simulink model "controller"  (Simulink 8.3)
settings: Solver=FixedStepDiscrete  StartTime=0.0  StopTime=simulationTime  FixedStep=Ts  RelTol=1e-3
InitFcn:
  | initBalancingController_with_opt_of_tau;
values from neighbouring files (symbols this model uses):
  noOscillationTime = 0    [initBalancingController_with_opt_of_tau.m]    (also in initBalancingOptTau.m)
  number_of_feet_on_ground = 2    [initBalancingController_with_opt_of_tau.m]    (also in initBalancingOptTau.m)
  Ts = 0.01    [initBalancingController_with_opt_of_tau.m]    (also in initBalancingOptTau.m)
undefined symbols (not defined in the file or in its folder): amplitudesOscillationsOnOneFoot, dampings, directionOfOscillation, DiscIntNeverNeededParam, frequenciesOscillationsOnOneFoot, gainMomentum, gainsDCOM, gainsICOM, gainsPCOM, impedances, impedencesSat, increasingRatesImp, integralGains, qTildeMax, referenceParams, ROBOT_DOF, ROBOT_DOF_FOR_SIMULINK, satIntegral
undefined symbols (not defined in the file): localName, robotName
libraries: WBCLibrary x38
settings Model: Creator=daniele  LastModifiedBy=daniele
settings DataIOCC: SignalLoggingSaveFormat=Dataset
settings OptimizationCC: ExpressionDepthLimit=2147483647
settings DebuggingCC: FcnCallInpInsideContextMsg=EnableAllAsWarning
settings SFSimCC: SimParseCustomCode=off

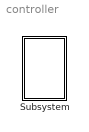
== system controller ==
  Subsystem : Subsystem  mask{robotName=robotName, Ts=Ts, localName=localName}
      mask prompts: robotName "robot name"; localName "module name"

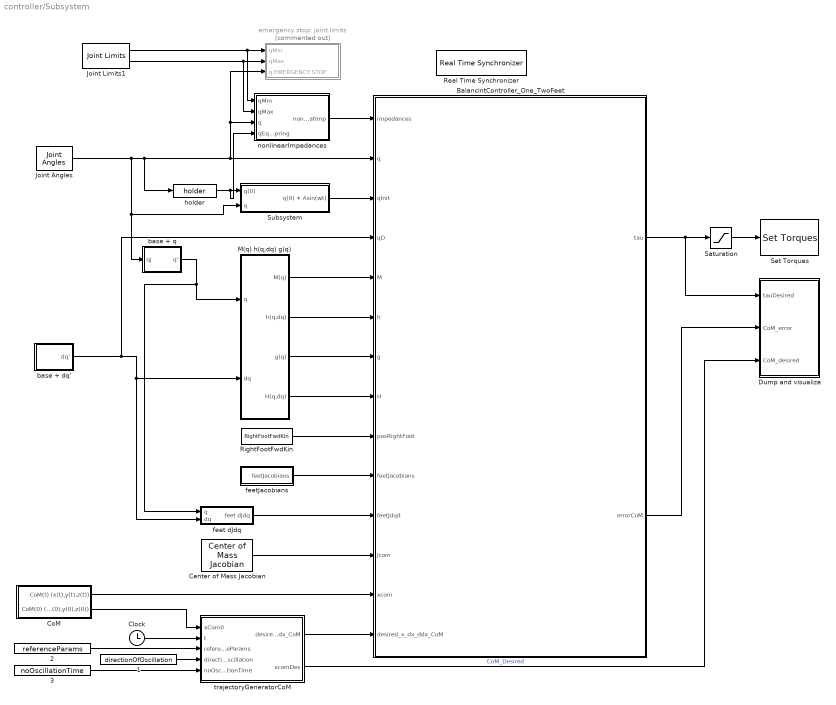
== system controller/Subsystem ==
  "    1" : Constant  Value=directionOfOscillation
  "    2" : Constant  Value=referenceParams
  "    3" : Constant  Value=noOscillationTime
  BalancintController_One_TwoFeet : Subsystem
  Center of Mass Jacobian : WBCLibrary/wholeBodyModel/Jacobians/Center of Mass Jacobian  robotName=robotName  localName=localName
  Clock : Clock
  "CoM " : Subsystem
  Dump and visualize : Subsystem
  Joint Angles : WBCLibrary/wholeBodyStates/Joint Angles  robotName=robotName  localName=localName
  Joint Limits1 : WBCLibrary/wholeBodyModel/Joint Limits  robotName=robotName  localName=localName
  M(q) h(q,dq) g(q) : Subsystem
  Real Time Synchronizer : WBCLibrary/Utilities/Real Time Synchronizer  Priority=-10  threadPeriod=Ts
  RightFootFwdKin : WBCLibrary/wholeBodyModel/Forward Kinematics/RightFootFwdKin  robotName=robotName  localName=localName
  Saturation : Saturate  UpperLimit=24  LowerLimit=-24
  Set Torques : WBCLibrary/wholeBodyActuators/Set Torques  val=6  robotName=robotName  localName=localName
  Subsystem : Subsystem
  base + dq' : Subsystem
  base + q : Subsystem
  emergency stop: joint limits : Subsystem  Commented=on
  feet dJdq : Subsystem
  feetJacobians : Subsystem
  "holder " : WBCLibrary/Utilities/holder 
  nonlinearImpedances : Subsystem
  trajectoryGeneratorCoM : MATLAB Function  TreatAsAtomicUnit=on
  wires:
  trajectoryGeneratorCoM/1(desired_x_dx_ddx_CoM) -> BalancintController_One_TwoFeet/14(desired_x_dx_ddx_CoM)
  "CoM "/2(CoM(0) (x(0),y(0),z(0))) -> trajectoryGeneratorCoM/1(xCom0)
  RightFootFwdKin/1 -> BalancintController_One_TwoFeet/9(posRightFoot)
  base + q/1(q') -> feet dJdq/1(q), M(q) h(q,dq) g(q)/1(q)
  M(q) h(q,dq) g(q)/3(g(q)) -> BalancintController_One_TwoFeet/7(g)
  M(q) h(q,dq) g(q)/4(H(q,dq)) -> BalancintController_One_TwoFeet/8(H)
  Center of Mass Jacobian/1 -> BalancintController_One_TwoFeet/12(Jcom)
  feetJacobians/1(feetJacobians) -> BalancintController_One_TwoFeet/10(feetJacobians)
  feet dJdq/1(feet dJdq) -> BalancintController_One_TwoFeet/11(feetJdqd)
  "holder "/1 -> nonlinearImpedances/4(qEquSpring), Subsystem/1(q(0))
  "CoM "/1(CoM(t) (x(t),y(t),z(t))) -> BalancintController_One_TwoFeet/13(xcom)
  base + dq'/1(dq') -> BalancintController_One_TwoFeet/4(qD), feet dJdq/2(dq), M(q) h(q,dq) g(q)/2(dq)
  M(q) h(q,dq) g(q)/1(M(q)) -> BalancintController_One_TwoFeet/5(M)
  M(q) h(q,dq) g(q)/2(h(q,dq)) -> BalancintController_One_TwoFeet/6(h)
  BalancintController_One_TwoFeet/1(tau) -> Saturation/1, Dump and visualize/1(tauDesired)
  "    2"/1 -> trajectoryGeneratorCoM/3(referenceParams)
  Clock/1 -> trajectoryGeneratorCoM/2(t)
  nonlinearImpedances/1(nonLinSatImp) -> BalancintController_One_TwoFeet/1(impedances)
  Joint Limits1/1 -> emergency stop: joint limits/1(qMin), nonlinearImpedances/1(qMin)
  Joint Limits1/2 -> emergency stop: joint limits/2(qMax), nonlinearImpedances/2(qMax)
  Joint Angles/1 -> Subsystem/2(q), base + q/1(qj), nonlinearImpedances/3(q), emergency stop: joint limits/3(q EMERGENCY STOP), BalancintController_One_TwoFeet/2(q), "holder "/1
  "    1"/1 -> trajectoryGeneratorCoM/4(directionOfOscillation)
  "    3"/1 -> trajectoryGeneratorCoM/5(noOscillationTime)
  Subsystem/1(q(0) + Asin(wt)) -> BalancintController_One_TwoFeet/3(qInit)
  BalancintController_One_TwoFeet/2(errorCoM) -> Dump and visualize/2(CoM_error)
  trajectoryGeneratorCoM/2(xcomDes) -> Dump and visualize/3(CoM_desired)  "CoM_Desired"
  Saturation/1 -> Set Torques/1

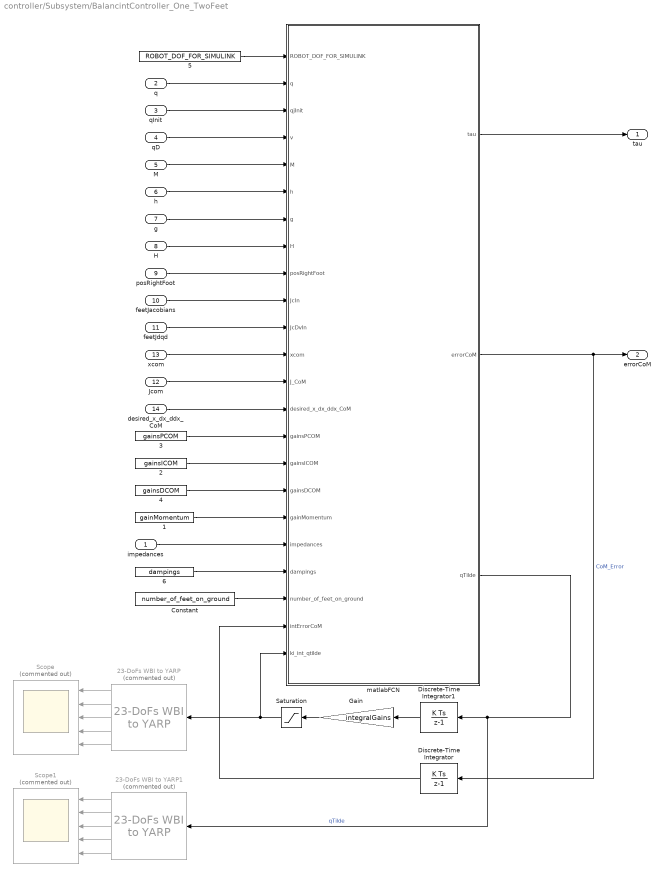
== system controller/Subsystem/BalancintController_One_TwoFeet ==
  impedances : Inport
  q : Inport  Port=2
  qInit : Inport  Port=3
  qD : Inport  Port=4
  M : Inport  Port=5
  h : Inport  Port=6
  g : Inport  Port=7
  H : Inport  Port=8
  posRightFoot : Inport  Port=9
  feetJacobians : Inport  Port=10
  feetJdqd : Inport  Port=11
  Jcom : Inport  Port=12
  xcom : Inport  Port=13
  desired_x_dx_ddx_CoM : Inport  Port=14
  "    1" : Constant  Value=gainMomentum
  "    2" : Constant  Value=gainsICOM
  "    3" : Constant  Value=gainsPCOM
  "    4" : Constant  Value=gainsDCOM
  "    5" : Constant  Value=ROBOT_DOF_FOR_SIMULINK
  "    6" : Constant  Value=dampings
  23-DoFs WBI to YARP : WBCLibrary/Utilities/23-DoFs WBI to YARP  Commented=on
  23-DoFs WBI to YARP1 : WBCLibrary/Utilities/23-DoFs WBI to YARP  Commented=on
  Constant : Constant  Value=number_of_feet_on_ground
  Discrete-Time Integrator : DiscreteIntegrator  InitialCondition=[0 0 0]  SampleTime=Ts  ICPrevOutput=DiscIntNeverNeededParam  ICPrevScaledInput=DiscIntNeverNeededParam
  Discrete-Time Integrator1 : DiscreteIntegrator  InitialCondition=zeros(ROBOT_DOF,1)  SampleTime=Ts  ICPrevOutput=DiscIntNeverNeededParam  ICPrevScaledInput=DiscIntNeverNeededParam
  Gain : Gain  Gain=integralGains
  Saturation : Saturate  UpperLimit=satIntegral  LowerLimit=-satIntegral
  Scope : Scope  Commented=on  NumInputPorts=5
      settings: ShowLegends=on  YMin=-5~-5~-5~-5~-5  YMax=5~5~5~5~5
  Scope1 : Scope  Commented=on  NumInputPorts=5
      settings: ShowLegends=on  YMin=-5~-5~-5~-5~-5  YMax=5~5~5~5~5  SaveName=ScopeData2
  matlabFCN : MATLAB Function  TreatAsAtomicUnit=on
  tau : Outport
  errorCoM : Outport  Port=2
  wires:
  q/1 -> matlabFCN/2(q)
  qInit/1 -> matlabFCN/3(qjInit)
  qD/1 -> matlabFCN/4(v)
  M/1 -> matlabFCN/5(M)
  h/1 -> matlabFCN/6(h)
  g/1 -> matlabFCN/7(g)
  H/1 -> matlabFCN/8(H)
  posRightFoot/1 -> matlabFCN/9(posRightFoot)
  feetJacobians/1 -> matlabFCN/10(JcIn)
  feetJdqd/1 -> matlabFCN/11(JcDvIn)
  xcom/1 -> matlabFCN/12(xcom)
  Jcom/1 -> matlabFCN/13(J_CoM)
  desired_x_dx_ddx_CoM/1 -> matlabFCN/14(desired_x_dx_ddx_CoM)
  impedances/1 -> matlabFCN/19(impedances)
  "    3"/1 -> matlabFCN/15(gainsPCOM)
  "    1"/1 -> matlabFCN/18(gainMomentum)
  "    2"/1 -> matlabFCN/16(gainsICOM)
  "    4"/1 -> matlabFCN/17(gainsDCOM)
  matlabFCN/1(tau) -> tau/1
  Constant/1 -> matlabFCN/21(number_of_feet_on_ground)
  "    5"/1 -> matlabFCN/1(ROBOT_DOF_FOR_SIMULINK)
  "    6"/1 -> matlabFCN/20(dampings)
  Discrete-Time Integrator/1 -> matlabFCN/22(intErrorCoM)
  matlabFCN/2(errorCoM) -> errorCoM/1, Discrete-Time Integrator/1  "CoM_Error"
  Discrete-Time Integrator1/1 -> Gain/1
  23-DoFs WBI to YARP/5 -> Scope/5
  23-DoFs WBI to YARP/1 -> Scope/1
  23-DoFs WBI to YARP/4 -> Scope/4
  23-DoFs WBI to YARP/2 -> Scope/2
  23-DoFs WBI to YARP/3 -> Scope/3
  matlabFCN/3(qTilde) -> 23-DoFs WBI to YARP1/1, Discrete-Time Integrator1/1  "qTilde"
  Gain/1 -> Saturation/1
  Saturation/1 -> 23-DoFs WBI to YARP/1, matlabFCN/23(ki_int_qtilde)
  23-DoFs WBI to YARP1/5 -> Scope1/5
  23-DoFs WBI to YARP1/1 -> Scope1/1
  23-DoFs WBI to YARP1/4 -> Scope1/4
  23-DoFs WBI to YARP1/2 -> Scope1/2
  23-DoFs WBI to YARP1/3 -> Scope1/3

== system controller/Subsystem/CoM  ==
  "COMFwdKin " : WBCLibrary/wholeBodyModel/Forward Kinematics/COMFwdKin   robotName=robotName  localName=localName
  "CoM6D ->  CoMXYZ" : Selector  InputPortWidth=7  Indices=[1 2 3]
  "holder " : WBCLibrary/Utilities/holder 
  CoM(t) (x(t),y(t),z(t)) : Outport
  CoM(0) (x(0),y(0),z(0)) : Outport  Port=2
  wires:
  "COMFwdKin "/1 -> "CoM6D ->  CoMXYZ"/1
  "CoM6D ->  CoMXYZ"/1 -> "holder "/1, CoM(t) (x(t),y(t),z(t))/1
  "holder "/1 -> CoM(0) (x(0),y(0),z(0))/1

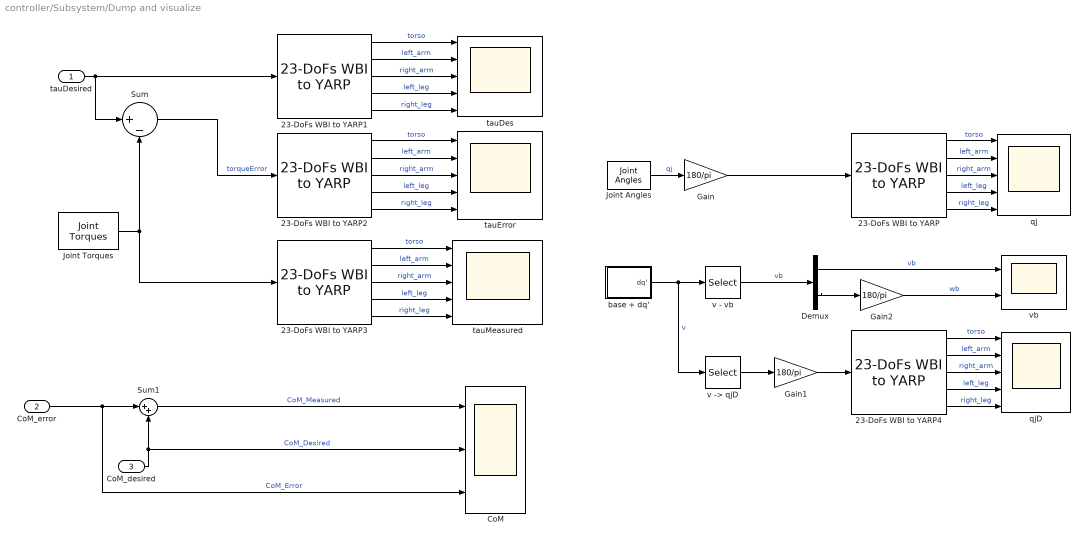
== system controller/Subsystem/Dump and visualize ==
  tauDesired : Inport
  CoM_error : Inport  Port=2
  CoM_desired : Inport  Port=3
  23-DoFs WBI to YARP{,1..4} (5 alike) : WBCLibrary/Utilities/23-DoFs WBI to YARP
  CoM : Scope  NumInputPorts=3
      settings: ShowLegends=on  TimeRange=400  YMin=-0.2~-0.2~-0.006  YMax=0.5~0.5~0.004  SaveName=CoM_data
  Demux : Demux  Outputs=2
  Gain : Gain  Gain=180/pi
  Gain1 : Gain  Gain=180/pi
  Gain2 : Gain  Gain=180/pi
  Joint Angles : WBCLibrary/wholeBodyStates/Joint Angles  robotName=robotName  localName=localName
  Joint Torques : WBCLibrary/wholeBodyStates/Joint Torques  robotName=robotName  localName=localName
  Sum : Sum  Inputs=|+-
  Sum1 : Sum  Inputs=|++
  base + dq' : Subsystem
  qj : Scope  NumInputPorts=5
      settings: ShowLegends=on  TimeRange=40  YMin=-10~-50~-50~-20~-40  YMax=10~100~100~40~40  SaveName=qj_and_v
  qjD : Scope  NumInputPorts=5
      settings: ShowLegends=on  TimeRange=40  YMin=-15~-10~-20~-20~-20  YMax=20~10~30~20~20  SaveName=qj_and_v1
  tauDes : Scope  NumInputPorts=5
      settings: ShowLegends=on  TimeRange=14  YMin=-20~-3~-3~-8~-10  YMax=10~3~3~4~10  SaveName=tauDes
  tauError : Scope  NumInputPorts=5
      settings: ShowLegends=on  TimeRange=90  YMin=-3~-6~-5~-4~-4  YMax=3~6~5~4~6  SaveName=tauError
  tauMeasured : Scope  NumInputPorts=5
      settings: ShowLegends=on  TimeRange=14  YMin=-15~-8~-5~-8~-10  YMax=10~4~5~6~10  SaveName=tauMeasured
  v - vb : Selector  InputPortWidth=ROBOT_DOF+6  Indices=[1:6]
  "v -> qjD" : Selector  InputPortWidth=ROBOT_DOF+6  Indices=[7:ROBOT_DOF+6]
  vb : Scope  NumInputPorts=2
      settings: ShowLegends=on  TimeRange=40  YMin=-0.08~-10  YMax=0.08~10  SaveName=qj_and_v2
  wires:
  CoM_error/1 -> CoM/3, Sum1/1  "CoM_Error"
  tauDesired/1 -> Sum/1, 23-DoFs WBI to YARP1/1
  Joint Torques/1 -> 23-DoFs WBI to YARP3/1, Sum/2
  CoM_desired/1 -> Sum1/2, CoM/2  "CoM_Desired"
  Sum1/1 -> CoM/1  "CoM_Measured"
  base + dq'/1(dq') -> "v -> qjD"/1, v - vb/1  "v"
  Joint Angles/1 -> Gain/1  "qj"
  Gain/1 -> 23-DoFs WBI to YARP/1
  23-DoFs WBI to YARP/5 -> qj/5  "right_leg"
  23-DoFs WBI to YARP/1 -> qj/1  "torso"
  23-DoFs WBI to YARP/2 -> qj/2  "left_arm"
  23-DoFs WBI to YARP/4 -> qj/4  "left_leg"
  23-DoFs WBI to YARP/3 -> qj/3  "right_arm"
  23-DoFs WBI to YARP1/5 -> tauDes/5  "right_leg"
  23-DoFs WBI to YARP1/1 -> tauDes/1  "torso"
  23-DoFs WBI to YARP1/2 -> tauDes/2  "left_arm"
  23-DoFs WBI to YARP1/4 -> tauDes/4  "left_leg"
  23-DoFs WBI to YARP1/3 -> tauDes/3  "right_arm"
  23-DoFs WBI to YARP2/5 -> tauError/5  "right_leg"
  23-DoFs WBI to YARP2/1 -> tauError/1  "torso"
  23-DoFs WBI to YARP2/2 -> tauError/2  "left_arm"
  23-DoFs WBI to YARP2/4 -> tauError/4  "left_leg"
  23-DoFs WBI to YARP2/3 -> tauError/3  "right_arm"
  Sum/1 -> 23-DoFs WBI to YARP2/1  "torqueError"
  23-DoFs WBI to YARP3/5 -> tauMeasured/5  "right_leg"
  23-DoFs WBI to YARP3/1 -> tauMeasured/1  "torso"
  23-DoFs WBI to YARP3/2 -> tauMeasured/2  "left_arm"
  23-DoFs WBI to YARP3/4 -> tauMeasured/4  "left_leg"
  23-DoFs WBI to YARP3/3 -> tauMeasured/3  "right_arm"
  23-DoFs WBI to YARP4/5 -> qjD/5  "right_leg"
  23-DoFs WBI to YARP4/1 -> qjD/1  "torso"
  23-DoFs WBI to YARP4/2 -> qjD/2  "left_arm"
  23-DoFs WBI to YARP4/4 -> qjD/4  "left_leg"
  23-DoFs WBI to YARP4/3 -> qjD/3  "right_arm"
  "v -> qjD"/1 -> Gain1/1
  v - vb/1 -> Demux/1  "vb"
  Demux/1 -> vb/1  "vb"
  Demux/2 -> Gain2/1
  Gain1/1 -> 23-DoFs WBI to YARP4/1
  Gain2/1 -> vb/2  "wb"

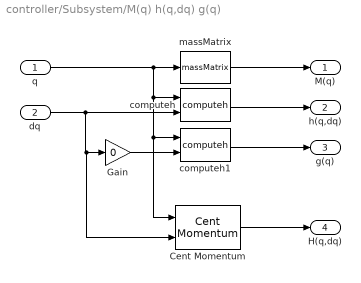
== system controller/Subsystem/M(q) h(q,dq) g(q) ==
  q : Inport
  dq : Inport  Port=2
  Cent Momentum : WBCLibrary/wholeBodyModel/Dynamics/Cent Momentum  robotName=robotName  localName=localName
  Gain : Gain  Gain=0
  computeh : WBCLibrary/wholeBodyModel/Dynamics/computeh  val=7  robotname=robotName  localname=localName
  computeh1 : WBCLibrary/wholeBodyModel/Dynamics/computeh  val=7  robotname=robotName  localname=localName
  massMatrix : WBCLibrary/wholeBodyModel/Dynamics/massMatrix  val=8  robotname=robotName  localname=localName
  M(q) : Outport
  h(q,dq) : Outport  Port=2
  g(q) : Outport  Port=3
  H(q,dq) : Outport  Port=4
  wires:
  Gain/1 -> computeh1/2
  computeh1/1 -> g(q)/1
  computeh/1 -> h(q,dq)/1
  massMatrix/1 -> M(q)/1
  q/1 -> Cent Momentum/1, computeh1/1, computeh/1, massMatrix/1
  dq/1 -> Cent Momentum/2, Gain/1, computeh/2
  Cent Momentum/1 -> H(q,dq)/1

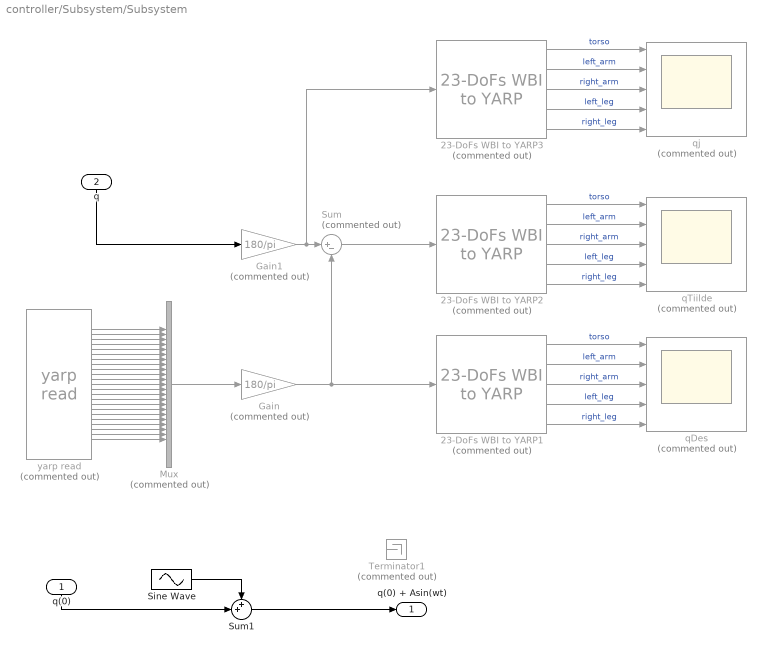
== system controller/Subsystem/Subsystem ==
  q(0) : Inport
  q : Inport  Port=2
  23-DoFs WBI to YARP1 : WBCLibrary/Utilities/23-DoFs WBI to YARP  Commented=on
  23-DoFs WBI to YARP2 : WBCLibrary/Utilities/23-DoFs WBI to YARP  Commented=on
  23-DoFs WBI to YARP3 : WBCLibrary/Utilities/23-DoFs WBI to YARP  Commented=on
  Gain : Gain  Commented=on  Gain=180/pi
  Gain1 : Gain  Commented=on  Gain=180/pi
  Mux : Mux  Commented=on  Inputs=23
  Sine Wave : Sin  Amplitude=amplitudesOscillationsOnOneFoot*pi/180  Frequency=frequenciesOscillationsOnOneFoot*2*pi  SampleTime=0
  Sum : Sum  Commented=on  Inputs=|+-
  Sum1 : Sum  Inputs=++|
  Terminator1 : Terminator  Commented=on
  qDes : Scope  Commented=on  NumInputPorts=5
      settings: ShowLegends=on  TimeRange=14  YMin=-20~-4~-4~-8~-10  YMax=10~4~4~4~10  SaveName=tauDes1
  qTiilde : Scope  Commented=on  NumInputPorts=5
      settings: ShowLegends=on  TimeRange=14  YMin=-20~-4~-4~-8~-10  YMax=10~4~4~4~10  SaveName=tauDes2
  qj : Scope  Commented=on  NumInputPorts=5
      settings: ShowLegends=on  TimeRange=14  YMin=-20~-4~-4~-8~-10  YMax=10~4~4~4~10  SaveName=tauDes3
  yarp read : WBCLibrary/Utilities/yarp read  Commented=on  from=['/trajGenY2/qdes:o']  to='...'  num=23  blocking=off  timestamp=off  autoconnect=on
  q(0) + Asin(wt) : Outport
  wires:
  q(0)/1 -> Sum1/2
  Sine Wave/1 -> Sum1/1
  Mux/1 -> Gain/1
  Gain/1 -> 23-DoFs WBI to YARP1/1, Sum/2
  q/1 -> Gain1/1
  Sum/1 -> 23-DoFs WBI to YARP2/1
  yarp read/18 -> Mux/18
  yarp read/16 -> Mux/16
  yarp read/21 -> Mux/21
  yarp read/23 -> Mux/23
  yarp read/22 -> Mux/22
  yarp read/17 -> Mux/17
  yarp read/19 -> Mux/19
  yarp read/20 -> Mux/20
  yarp read/4 -> Mux/4
  yarp read/5 -> Mux/5
  yarp read/6 -> Mux/6
  yarp read/7 -> Mux/7
  yarp read/8 -> Mux/8
  yarp read/9 -> Mux/9
  yarp read/10 -> Mux/10
  yarp read/11 -> Mux/11
  yarp read/12 -> Mux/12
  yarp read/13 -> Mux/13
  yarp read/14 -> Mux/14
  yarp read/3 -> Mux/3
  yarp read/1 -> Mux/1
  yarp read/2 -> Mux/2
  yarp read/15 -> Mux/15
  Gain1/1 -> 23-DoFs WBI to YARP3/1, Sum/1
  23-DoFs WBI to YARP1/5 -> qDes/5  "right_leg"
  23-DoFs WBI to YARP1/1 -> qDes/1  "torso"
  23-DoFs WBI to YARP1/2 -> qDes/2  "left_arm"
  23-DoFs WBI to YARP1/4 -> qDes/4  "left_leg"
  23-DoFs WBI to YARP1/3 -> qDes/3  "right_arm"
  23-DoFs WBI to YARP2/5 -> qTiilde/5  "right_leg"
  23-DoFs WBI to YARP2/1 -> qTiilde/1  "torso"
  23-DoFs WBI to YARP2/2 -> qTiilde/2  "left_arm"
  23-DoFs WBI to YARP2/4 -> qTiilde/4  "left_leg"
  23-DoFs WBI to YARP2/3 -> qTiilde/3  "right_arm"
  23-DoFs WBI to YARP3/5 -> qj/5  "right_leg"
  23-DoFs WBI to YARP3/1 -> qj/1  "torso"
  23-DoFs WBI to YARP3/2 -> qj/2  "left_arm"
  23-DoFs WBI to YARP3/4 -> qj/4  "left_leg"
  23-DoFs WBI to YARP3/3 -> qj/3  "right_arm"
  Sum1/1 -> q(0) + Asin(wt)/1

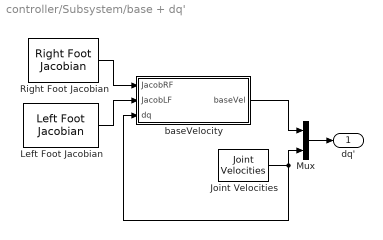
== system controller/Subsystem/base + dq' ==
  Joint Velocities : WBCLibrary/wholeBodyStates/Joint Velocities  robotName=robotName  localName=localName
  Left Foot Jacobian : WBCLibrary/wholeBodyModel/Jacobians/Left Foot Jacobian  robotName=robotName  localName=localName
  Mux : Mux  Inputs=2
  Right Foot Jacobian : WBCLibrary/wholeBodyModel/Jacobians/Right Foot Jacobian  robotName=robotName  localName=localName
  baseVelocity : Subsystem  AncestorBlock=WBCLibrary/Utilities/baseVelocity  mask(baseVelocity){}
      mask help: This block computes the velocity of the floating base of a bipedal robot
  dq' : Outport
  wires:
  Left Foot Jacobian/1 -> baseVelocity/2(JacobLF)
  Right Foot Jacobian/1 -> baseVelocity/1(JacobRF)
  baseVelocity/1(baseVel) -> Mux/1
  Joint Velocities/1 -> baseVelocity/3(dq), Mux/2
  Mux/1 -> dq'/1

== system controller/Subsystem/base + q ==
  qj : Inport
  Constant1 : Constant  Value=zeros(16,1)
  Mux : Mux  Inputs=2
  q' : Outport
  wires:
  Mux/1 -> q'/1
  qj/1 -> Mux/2
  Constant1/1 -> Mux/1

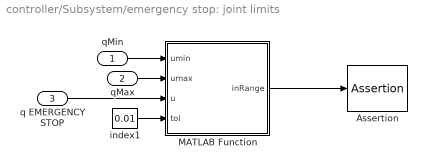
== system controller/Subsystem/emergency stop: joint limits ==
  qMin : Inport
  qMax : Inport  Port=2
  q EMERGENCY STOP : Inport  Port=3
  Assertion : Assertion
  MATLAB Function : MATLAB Function  TreatAsAtomicUnit=on
  index1 : Constant  Value=0.01  VectorParams1D=off
  wires:
  qMin/1 -> MATLAB Function/1(umin)
  qMax/1 -> MATLAB Function/2(umax)
  index1/1 -> MATLAB Function/4(tol)
  q EMERGENCY STOP/1 -> MATLAB Function/3(u)
  MATLAB Function/1(inRange) -> Assertion/1

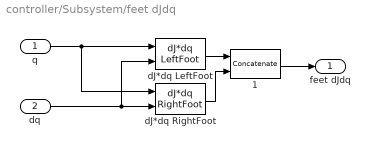
== system controller/Subsystem/feet dJdq ==
  q : Inport
  dq : Inport  Port=2
  " 1" : Concatenate  Mode=Multidimensional array
  dJ*dq LeftFoot : WBCLibrary/wholeBodyModel/Dynamics/dJ*dq LeftFoot  val=9  robotName=robotName  localName=localName
  dJ*dq RightFoot : WBCLibrary/wholeBodyModel/Dynamics/dJ*dq RightFoot  val=9  robotName=robotName  localName=localName
  feet dJdq : Outport
  wires:
  dJ*dq LeftFoot/1 -> " 1"/1
  dJ*dq RightFoot/1 -> " 1"/2
  " 1"/1 -> feet dJdq/1
  q/1 -> dJ*dq RightFoot/1, dJ*dq LeftFoot/1
  dq/1 -> dJ*dq LeftFoot/2, dJ*dq RightFoot/2

== system controller/Subsystem/feetJacobians ==
  " " : Concatenate  Mode=Multidimensional array
  Left Foot Jacobian : WBCLibrary/wholeBodyModel/Jacobians/Left Foot Jacobian  robotName=robotName  localName=localName
  Right Foot Jacobian : WBCLibrary/wholeBodyModel/Jacobians/Right Foot Jacobian  robotName=robotName  localName=localName
  feetJacobians : Outport
  wires:
  Left Foot Jacobian/1 -> " "/1
  Right Foot Jacobian/1 -> " "/2
  " "/1 -> feetJacobians/1

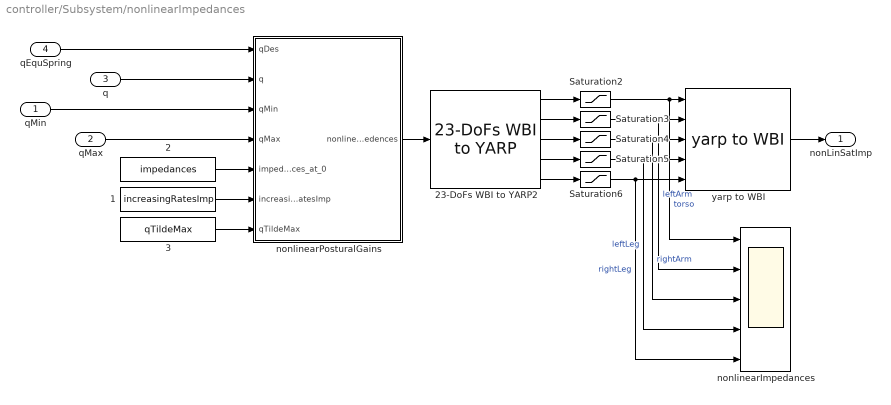
== system controller/Subsystem/nonlinearImpedances ==
  qMin : Inport
  qMax : Inport  Port=2
  q : Inport  Port=3
  qEquSpring : Inport  Port=4
  "    1" : Constant  Value=increasingRatesImp
  "    2" : Constant  Value=impedances
  "    3" : Constant  Value=qTildeMax
  23-DoFs WBI to YARP2 : WBCLibrary/Utilities/23-DoFs WBI to YARP
  Saturation2 : Saturate  UpperLimit=impedencesSat(1)  LowerLimit=0  SampleTime=Ts
  Saturation3 : Saturate  UpperLimit=impedencesSat(2)  LowerLimit=0  SampleTime=Ts
  Saturation4 : Saturate  UpperLimit=impedencesSat(2)  LowerLimit=0  SampleTime=Ts
  Saturation5 : Saturate  UpperLimit=impedencesSat(3)  LowerLimit=0  SampleTime=Ts
  Saturation6 : Saturate  UpperLimit=impedencesSat(3)  LowerLimit=0  SampleTime=Ts
  nonlinearImpedances : Scope  NumInputPorts=5
      settings: ShowLegends=on  TimeRange=40  YMin=-50~-50~-50~0~0  YMax=50~50~50~1000~1000
  "nonlinearPosturalGains " : MATLAB Function  TreatAsAtomicUnit=on
  yarp to WBI : WBCLibrary/Utilities/yarp to WBI
  nonLinSatImp : Outport
  wires:
  23-DoFs WBI to YARP2/1 -> Saturation2/1
  23-DoFs WBI to YARP2/2 -> Saturation3/1
  23-DoFs WBI to YARP2/3 -> Saturation4/1
  23-DoFs WBI to YARP2/5 -> Saturation6/1
  "nonlinearPosturalGains "/1(nonlinearImpedences) -> 23-DoFs WBI to YARP2/1
  qEquSpring/1 -> "nonlinearPosturalGains "/1(qDes)
  qMin/1 -> "nonlinearPosturalGains "/3(qMin)
  qMax/1 -> "nonlinearPosturalGains "/4(qMax)
  "    2"/1 -> "nonlinearPosturalGains "/5(impedences_at_0)
  "    1"/1 -> "nonlinearPosturalGains "/6(increasingRatesImp)
  q/1 -> "nonlinearPosturalGains "/2(q)
  Saturation6/1 -> nonlinearImpedances/5, yarp to WBI/5  "rightLeg"
  Saturation4/1 -> nonlinearImpedances/3, yarp to WBI/3  "rightArm"
  Saturation5/1 -> nonlinearImpedances/4, yarp to WBI/4  "leftLeg"
  Saturation3/1 -> nonlinearImpedances/2, yarp to WBI/2  "leftArm"
  Saturation2/1 -> nonlinearImpedances/1, yarp to WBI/1  "torso"
  23-DoFs WBI to YARP2/4 -> Saturation5/1
  "    3"/1 -> "nonlinearPosturalGains "/7(qTildeMax)
  yarp to WBI/1 -> nonLinSatImp/1

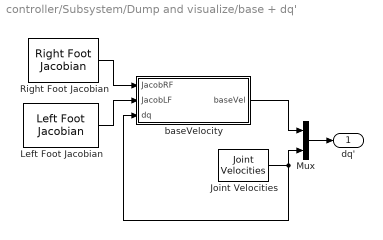
== system controller/Subsystem/Dump and visualize/base + dq' ==
  Joint Velocities : WBCLibrary/wholeBodyStates/Joint Velocities  robotName=robotName  localName=localName
  Left Foot Jacobian : WBCLibrary/wholeBodyModel/Jacobians/Left Foot Jacobian  robotName=robotName  localName=localName
  Mux : Mux  Inputs=2
  Right Foot Jacobian : WBCLibrary/wholeBodyModel/Jacobians/Right Foot Jacobian  robotName=robotName  localName=localName
  baseVelocity : Subsystem  AncestorBlock=WBCLibrary/Utilities/baseVelocity  mask(baseVelocity){}
      mask help: This block computes the velocity of the floating base of a bipedal robot
  dq' : Outport
  wires:
  Left Foot Jacobian/1 -> baseVelocity/2(JacobLF)
  Right Foot Jacobian/1 -> baseVelocity/1(JacobRF)
  baseVelocity/1(baseVel) -> Mux/1
  Joint Velocities/1 -> baseVelocity/3(dq), Mux/2
  Mux/1 -> dq'/1

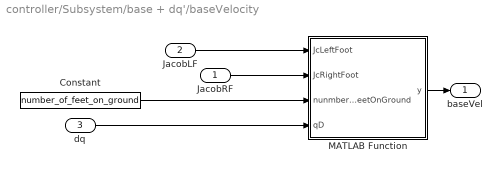
== system controller/Subsystem/base + dq'/baseVelocity ==
  JacobRF : Inport
  JacobLF : Inport  Port=2
  dq : Inport  Port=3
  Constant : Constant  Value=number_of_feet_on_ground
  MATLAB Function : MATLAB Function  TreatAsAtomicUnit=on
  baseVel : Outport
  wires:
  JacobLF/1 -> MATLAB Function/1(JcLeftFoot)
  JacobRF/1 -> MATLAB Function/2(JcRightFoot)
  MATLAB Function/1(y) -> baseVel/1
  dq/1 -> MATLAB Function/4(qD)
  Constant/1 -> MATLAB Function/3(nunmberOfFeetOnGround)

== system controller/Subsystem/Dump and visualize/base + dq'/baseVelocity ==
  JacobRF : Inport
  JacobLF : Inport  Port=2
  dq : Inport  Port=3
  Constant : Constant  Value=number_of_feet_on_ground
  MATLAB Function : MATLAB Function  TreatAsAtomicUnit=on
  baseVel : Outport
  wires:
  JacobLF/1 -> MATLAB Function/1(JcLeftFoot)
  JacobRF/1 -> MATLAB Function/2(JcRightFoot)
  MATLAB Function/1(y) -> baseVel/1
  dq/1 -> MATLAB Function/4(qD)
  Constant/1 -> MATLAB Function/3(nunmberOfFeetOnGround)

== matlab function Subsystem/trajectoryGeneratorCoM ==
  data: desired_x_dx_ddx_CoM output double; xCom0 input double; t input double; referenceParams input double; directionOfOscillation input double; noOscillationTime input double; xcomDes output double
function [desired_x_dx_ddx_CoM,xcomDes] = fcn(xCom0,t,referenceParams,directionOfOscillation,noOscillationTime)
%#codegen


if t > noOscillationTime
    A = referenceParams(1);
else
    A = 0;
end
f = referenceParams(2);

xcomDes    = xCom0 + A*sin(2*pi*f*t)*directionOfOscillation;
% xcomDes(1) =  xcomDes(1) + 0.01;
xDcomDes   =         A*2*pi*f*cos(2*pi*f*t)*directionOfOscillation;
xDDcomDes  =        -A*(2*pi*f)^2*sin(2*pi*f*t)*directionOfOscillation;

desired_x_dx_ddx_CoM = [xcomDes,xDcomDes,xDDcomDes];

== matlab function Subsystem/base + dq'/baseVelocity/MATLAB Function ==
  data: JcLeftFoot input double; JcRightFoot input double; nunmberOfFeetOnGround input double; y output double; qD input double
function y = fcn(JcLeftFoot,JcRightFoot,nunmberOfFeetOnGround,qD)
%#codegen
if nunmberOfFeetOnGround == 2
    Jc = [JcLeftFoot;JcRightFoot];
else
    Jc = JcLeftFoot;
end
y = -pinv(Jc(:,1:6))*Jc(:,7:end)*qD;

== matlab function Subsystem/BalancintController_One_TwoFeet/matlabFCN ==
  data: ROBOT_DOF_FOR_SIMULINK input double; q input double; tau output double; qjInit input double; v input double; M input double; h input double; g input double; H input double; posRightFoot input double; JcIn input double; JcDvIn input double; xcom input double; J_CoM input double; desired_x_dx_ddx_CoM input double; gainsPCOM input double; gainsICOM input double; gainsDCOM input double; gainMomentum input double; impedances input double; dampings input double; number_of_feet_on_ground input double; intErrorCoM input double; errorCoM output double; ki_int_qtilde input double; qTilde output double
function [tau,errorCoM,qTilde]   =  fcnQP_part1(ROBOT_DOF_FOR_SIMULINK,q,qjInit,v, M, h, g, H, posRightFoot, JcIn, JcDvIn, xcom,J_CoM, desired_x_dx_ddx_CoM, gainsPCOM,gainsICOM,gainsDCOM,gainMomentum, impedances,dampings, number_of_feet_on_ground,intErrorCoM,ki_int_qtilde)


ROBOT_DOF       = size(ROBOT_DOF_FOR_SIMULINK,1);
PINV_TOL        = 1e-5;
reg             = 0.01;
gravAcc         = 9.81;
m               = M(1,1);
Mb              = M(1:6,1:6);
Mbj             = M(1:6,7:end);
Mj              = M(7:end,7:end);

St              = [  zeros(6,ROBOT_DOF);
                   eye(ROBOT_DOF,ROBOT_DOF)];
grav            = [ zeros(2,1);
                   -m*gravAcc;
                    zeros(3,1)];
pos_rightFoot   = posRightFoot(1:3);

xDcom           = J_CoM(1:3,:)*v;
qD              = v(7:end);
xDDcomStar      = desired_x_dx_ddx_CoM(:,3) - gainsPCOM*(xcom - desired_x_dx_ddx_CoM(:,1)) - gainsICOM*intErrorCoM - gainsDCOM*(xDcom - desired_x_dx_ddx_CoM(:,2));
Pr              = pos_rightFoot - xcom; % Application point of the contact force on the right foot w.r.t. CoM

if  number_of_feet_on_ground == 1
        A  = [ eye(3),   zeros(3);
             -Sf(xcom),  eye(3)];
         Jc = JcIn(1:6,:);
         JcDv = JcDvIn(1:6);
else
        A  = [ eye(3),   zeros(3),eye(3), zeros(3);
             -Sf(xcom),  eye(3), Sf(Pr), eye(3) ];
         Jc = JcIn;
         JcDv = JcDvIn;
end        

JcMinv          = Jc/M;
JcMinvSt        = JcMinv*St;
JcMinvJct       = JcMinv*transpose(Jc);

pinvA         = pinv(        A, PINV_TOL);
% PInv_JcMinvSt = pinv( JcMinvSt, PINV_TOL);
PInv_JcMinvSt = JcMinvSt'/(JcMinvSt*JcMinvSt' + reg*eye(size(JcMinvSt,1)));
  
HDotDes  = [ m*xDDcomStar ;
            -gainMomentum*H(4:end)]; 
         
%% QP FOR TORQUE MINIMIZATION BASED ON arbitrary vector F0
% Maux = [     eye(3)     zeros(3,22)
%           zeros(22,3)      inv(Mj(4:end,4:end))];
%define tau_0 (the arbitrary vector)
N0_tau        = eye(ROBOT_DOF) - PInv_JcMinvSt*JcMinvSt;

mult_f_tau0   =  Mbj'/Mb*transpose(Jc(:,1:6))-transpose(Jc(:,7:end)); % multiplier of f in tau0
qTilde        =  q-qjInit;
n_tau0        =  h(7:end) -diag(impedances)*qTilde-ki_int_qtilde - Mbj'/Mb*h(1:6) -diag(dampings)*N0_tau*qD ; % additional terms in tau0 - Mj*(kPandD_Postural(1,:)'.*qTilde + kPandD_Postural(2,:)'.*qD) 
%

mult_f_tau    = N0_tau*mult_f_tau0  -PInv_JcMinvSt*JcMinvJct ;
n_tau         = PInv_JcMinvSt*(JcMinv*h-JcDv) + N0_tau*n_tau0;


% f desired is given as:
% f*   = pinvA*(HDotDes - grav)  + (I-pinvA*A) * f0
% f*   =           f_HDot        +     N0_f    * f0
f_HDot = pinvA*(HDotDes - grav);

% tau is given as:
% tau = (mult_f_tau*N0_f)* f0 + (n_tau+mult_f_tau*f_HDot)
% tau =        X_tau     * f0 +                   Y_tau

Y_tau         = n_tau + mult_f_tau*f_HDot;
tau           = Y_tau;
if number_of_feet_on_ground == 2
    N0_f          = eye(12,12)-pinvA*A;
    X_tau         = mult_f_tau*N0_f;
    f0            = -pinv(X_tau)*Y_tau;
    tau           = X_tau     * f0 +                   Y_tau;
end

errorCoM = xcom - desired_x_dx_ddx_CoM(:,1);

== matlab function Subsystem/emergency stop: joint limits/MATLAB Function ==
  data: umin input double; umax input double; u input double; inRange output double; tol input double
function inRange = checkRange(umin, umax, u, tol)
%#codegen

res = u < umin + tol | u > umax - tol;
res = sum(res);
if res==0
    inRange = 1;
else
    inRange = 0;
    u < umin + tol | u > umax - tol
end

== matlab function Subsystem/Dump and visualize/base + dq'/baseVelocity/MATLAB Function ==
  data: JcLeftFoot input double; JcRightFoot input double; nunmberOfFeetOnGround input double; y output double; qD input double
function y = fcn(JcLeftFoot,JcRightFoot,nunmberOfFeetOnGround,qD)
%#codegen
if nunmberOfFeetOnGround == 2
    Jc = [JcLeftFoot;JcRightFoot];
else
    Jc = JcLeftFoot;
end
y = -pinv(Jc(:,1:6))*Jc(:,7:end)*qD;

== matlab function Subsystem/nonlinearImpedances/nonlinearPosturalGains  ==
  data: qDes input double; nonlinearImpedences output double; q input double; qMin input double; qMax input double; impedences_at_0 input double; increasingRatesImp input double; qTildeMax input double
function nonlinearImpedences = fcn(qDes,q,qMin,qMax,impedences_at_0,increasingRatesImp,qTildeMax)
    %#codegen

    tp =  pi./(2*(qMax-qDes));
    tn = -pi./(2*(qMin-qDes));

    
    qTilde = q - qDes;
            
    nonlinearImpedences = (impedences_at_0   + increasingRatesImp.*tan(pi.*qTilde./(2*qTildeMax)).^2)';
%                                                increasingRatesImp.*tan((tp.*stepFcn(qTilde) + tn.*stepFcn(-qTilde)).*qTilde).^2)';
                                           
end

function y = stepFcn(x) 
   %#codegen
   y = x > 0; 
end
